simulink model "bai5"  (R2022b)
settings: Solver=ode4  StartTime=0.0  StopTime=40  FixedStep=0.001  RelTol=1e-3
undefined symbols (not defined in the file or in its folder): ki, kp
settings Model: Creator=ASUS  LastModifiedBy=ASUS

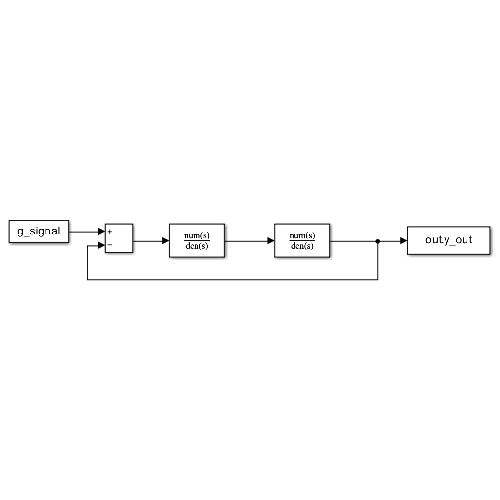
[thumbnail: Simulink's stored preview of the top-level diagram]
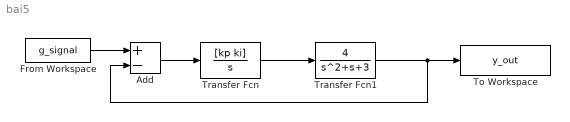
== system bai5 ==
  Add : Sum  Inputs=+-
  From Workspace : FromWorkspace  VariableName=g_signal
  To Workspace : ToWorkspace  VariableName=y_out  SaveFormat=Structure With Time  SampleTime=-1
  Transfer Fcn : TransferFcn  Numerator=[kp ki]  Denominator=[1 0]
  Transfer Fcn1 : TransferFcn  Numerator=[4]  Denominator=[1 1 3]
  wires:
  From Workspace/1 -> Add/1
  Add/1 -> Transfer Fcn/1
  Transfer Fcn/1 -> Transfer Fcn1/1
  Transfer Fcn1/1 -> Add/2, To Workspace/1
